simulink model "NonLinear_LQG"  (R2018a)
settings: Solver=VariableStepAuto  StartTime=0.0  StopTime=50.0  RelTol=1e-3
undefined symbols (not defined in the file): A, B, C, K
libraries: dspsrcs4 x1, peLuenbergerObserver x1
settings Model: Creator=kathp  LastModifiedBy=kathp

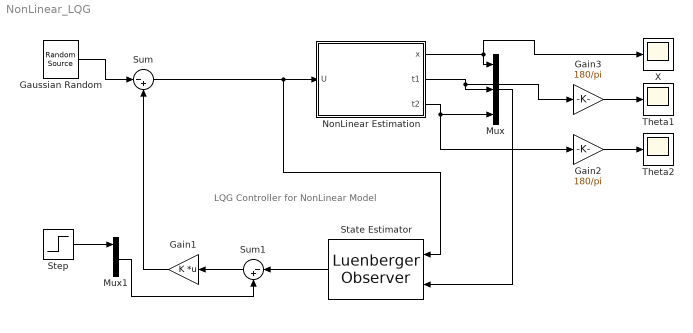
== system NonLinear_LQG ==
  note: LQG Controller for NonLinear Model
  Gain1 : Gain  Gain=K  Multiplication=Matrix(K*u)
  Gain2 : Gain  Gain=180/pi
  Gain3 : Gain  Gain=180/pi
  "Gaussian Random " : dspsrcs4/Random Source  SrcType=Gaussian  NormMethod=Ziggurat  CltLength=12  MinVal=0  MaxVal=0.5  MeanVal=0  VarVal=5  RepMode=Not repeatable  rawSeed=1  IsInherit=off  SampMode=Discrete  SampTime=1  SampFrame=1  DataType=Double  OutComplex=Real  OutputFrames=off
  Mux : Mux  Inputs=3
  Mux1 : Mux  Inputs=6
  "NonLinear Estimation " : Subsystem
  State Estimator : peLuenbergerObserver/Luenberger Observer  StateSpaceType=Continuous-time  Ad=A  Bd=B  Cd=C  Dd=[0;0;0]  A=A  B=B  C=C  D=[0;0;0]  ObserverDesign=Observer gain  Ld=L  DesiredEigenvalues=[-2.1 -2.32 -2.34 -2.36 -2.38 -3]  x0=[0;0;pi/10;0;pi/20;0]  Tsd=0.1  Ts=0.1
  Step : Step  SampleTime=0
  Sum : Sum  Inputs=|-+
  Sum1 : Sum  Inputs=|-+
  Theta1 : Scope
  Theta2 : Scope
  X : Scope
  wires:
  Mux/1 -> State Estimator/2
  Gain3/1 -> Theta1/1
  Gain2/1 -> Theta2/1
  "NonLinear Estimation "/3(t2) -> Mux/3, Gain2/1
  Sum/1 -> State Estimator/1, "NonLinear Estimation "/1(U)
  "NonLinear Estimation "/1(x) -> Mux/1, X/1
  "NonLinear Estimation "/2(t1) -> Mux/2, Gain3/1
  Gain1/1 -> Sum/2
  "Gaussian Random "/1 -> Sum/1
  Sum1/1 -> Gain1/1
  State Estimator/1 -> Sum1/1
  Step/1 -> Mux1/1
  Mux1/1 -> Sum1/2

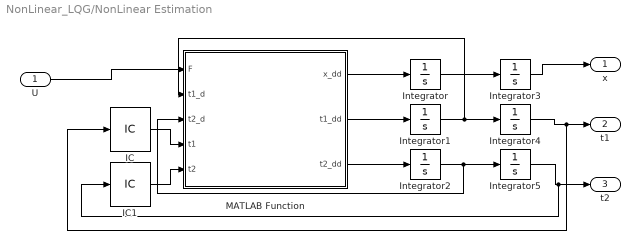
== system NonLinear_LQG/NonLinear Estimation  ==
  U : Inport
  IC : InitialCondition  Value=pi/10
  IC1 : InitialCondition  Value=pi/20
  Integrator : Integrator  UpperSaturationLimit=1000  LowerSaturationLimit=-1000
  Integrator1 : Integrator  UpperSaturationLimit=1000  LowerSaturationLimit=-1000
  Integrator2 : Integrator  UpperSaturationLimit=1000  LowerSaturationLimit=-1000
  Integrator3 : Integrator
  Integrator4 : Integrator
  Integrator5 : Integrator
  MATLAB Function : MATLAB Function  TreatAsAtomicUnit=on
  x : Outport
  t1 : Outport  Port=2
  t2 : Outport  Port=3
  wires:
  Integrator1/1 -> MATLAB Function/2(t1_d), Integrator4/1
  Integrator/1 -> Integrator3/1
  MATLAB Function/2(t1_dd) -> Integrator1/1
  MATLAB Function/3(t2_dd) -> Integrator2/1
  MATLAB Function/1(x_dd) -> Integrator/1
  Integrator2/1 -> MATLAB Function/3(t2_d), Integrator5/1
  Integrator4/1 -> IC/1, t1/1
  Integrator3/1 -> x/1
  Integrator5/1 -> IC1/1, t2/1
  U/1 -> MATLAB Function/1(F)
  IC/1 -> MATLAB Function/4(t1)
  IC1/1 -> MATLAB Function/5(t2)

== matlab function NonLinear_LQG/NonLinear Estimation /MATLAB Function ==
  data: F input; x_dd output; t1_d input; t2_d input; t1 input; t2 input; t1_dd output; t2_dd output
function [x_dd,t1_dd,t2_dd] = NonLinear_Estimation(F,t1_d,t2_d,t1,t2)

%% System Parameters
l1 = 20;
l2 = 10;
m1 = 100;
m2 = 100;
M = 1000;
g=9.8;

%% Variables
c1 = cos(t1);
c2 = cos(t2);
s1 = sin(t1);
s2 = sin(t2);

%% x_dd
x_dd = (F- (m1*l1*(t1_d^2)*(s1)) - (m2*l2*(t2_d^2)*(s2)) - m1*c1*s1*g - m2*c2*s2*g)/(M + m1*(s1^2) + m2*(s2^2));

%% t1_dd
t1_dd = (x_dd*c1 - g*s1)/l1;

%% t2_dd
t2_dd = (x_dd*c2 - g*s2)/l2;

end
